simulink library "robotlib"  (R2025a)
settings: Solver=ode45  StartTime=0.0  StopTime=10.0  RelTol=1e-3  EnableMultiTasking=on
undefined symbols (not defined in the file): coder, Count, Data, Data_SL_Info, Datatype, Encoding, Encoding_SL_Info, Fields, Fields_SL_Info, Header, Height, Name, Name_SL_Info, Offset, PointStep, ros, RowStep, Step, Width
libraries: $bdroot x1
(part 1 of 2)
settings Model: Creator=The MathWorks, Inc.  LastModifiedBy=The MathWorks, Inc.
settings SolverCC: AlgebraicLoopSolver=TrustRegion  MaxZcPerStep=1.0
settings DataIOCC: LimitDataPoints=on  SaveFormat=Array  ReturnWorkspaceOutputs=off
settings OptimizationCC: ReuseModelBlockBuffer=off  LifeSpan=inf
settings DebuggingCC: SolverPrmCheckMsg=warning  UnconnectedInputMsg=warning  UnconnectedOutputMsg=warning  UnconnectedLineMsg=warning  AllowSymbolicDim=off  PregeneratedLibrarySubsystemCodeDiagnostic=none  SubsystemReferenceDiagnosticForUnitTest=warning  SFUnexpectedBacktrackingDiag=warning  SFNoUnconditionalDefaultTransitionDiag=warning  SFExecutionAtInitializationDiag=none  ArithmeticOperatorsInVariantConditions=warning
settings HardwareCC: ProdBitPerPointer=32.0  ProdBitPerSizeT=32.0  ProdBitPerPtrDiffT=32.0  ProdLargestAtomicFloat=None  ProdIntDivRoundTo=Undefined  ProdEndianess=Unspecified  ProdWordSize=32.0  ProdHWDeviceType=32-bit Generic
settings ModelReferenceCC: EnableRefExpFcnMdlSchedulingChecks=on  PropagateSignalLabelsOutOfModel=off
settings SFSimCC: SimUseLocalCustomCode=off
settings RTWCC: RTWUseLocalCustomCode=off  GPUComputeCapability=3.5  DLArmComputeVersion=19.05
settings CodeAppCC: StateflowObjectComments=on
settings GRTTargetCC: TargetLangStandard=C89/C90 (ANSI)
settings ConfigComp: CovScope=ReferencedModels  CovMetricSettings=dw  CovSaveCumulativeToWorkspaceVar=on  CovSaveSingleToWorkspaceVar=on  CovExternalEMLEnable=off  CovSFcnEnable=off

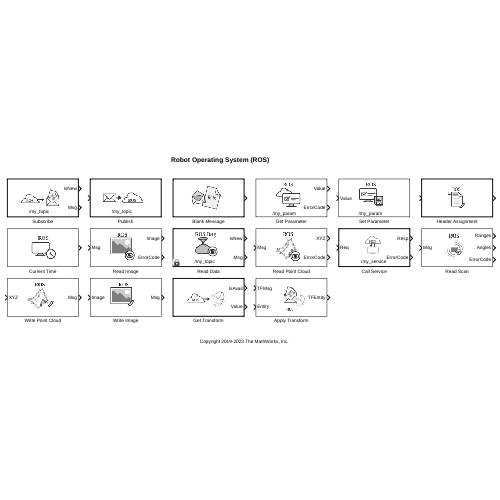
[thumbnail: Simulink's stored preview of the top-level diagram]
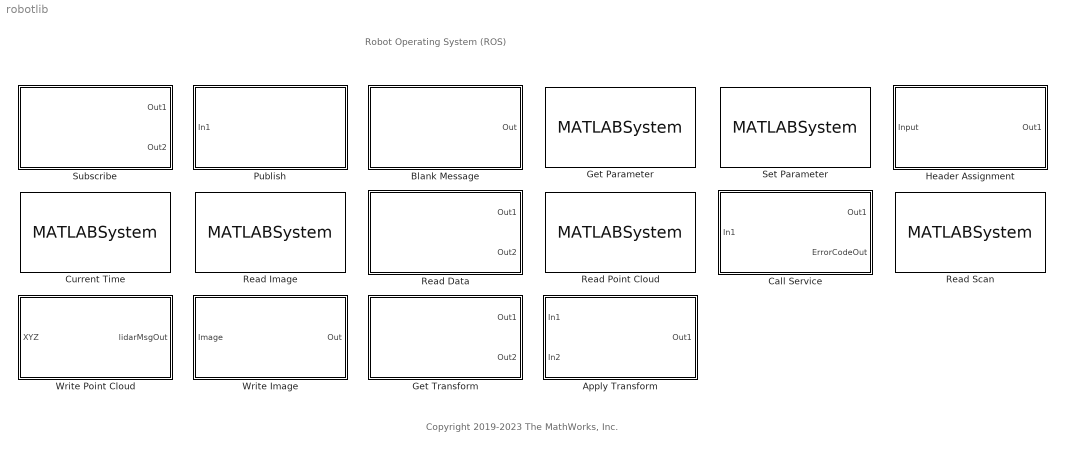
== system robotlib ==
  note: Copyright 2019-2023 The MathWorks, Inc.
  note: Robot Operating System (ROS)
  Apply Transform : Subsystem  InitFcn=ros.slros.internal.block.errorIfBlocksConflict(bdroot(gcb));  SystemSampleTime=SampleTime  mask(ros.slroscpp.internal.block.ApplyTransform){EntityMsgType=geometry_msgs/QuaternionStamped, SampleTime=-1}
      mask prompts: EntityMsgType "ros:slros:blockmask:EntityMsgPrompt"; SampleTime "Simulink:blkprm_prompts:AllBlksSampleTime"
      mask help: ros:slros:blockmask:ApplyTransformDescription
      mask init:
      | ros.slros.internal.block.ApplyTransformBlockMask.dispatch('maskInitialize', gcb);
      settings: ModelCloseFcn=ros.slros.internal.block.ApplyTransformBlockMask.dispatch('modelCloseFcn', gcb);
      mask Help: eval('ros.slros.internal.helpview(''rosApplyTransformBlock'')');
      mask TypeOptions EntityMsgType: ApplyTransform/EntityMsgType
      mask Callback EntityMsgType: ros.slros.internal.block.ApplyTransformBlockMask.dispatch('entityMsgTypeSelect', gcb);
      mask TypeOptions SampleTime: SystemSampleTime
      mask DialogControl DescGroupVar Prompt: ros:slros:blockmask:ApplyTransformMaskTitle
      mask DialogControl EntityMsgType Prompt: Entity message type:
      mask DialogControl SampleTime Prompt: Sample time (-1 for inherited):
      mask Display:
      | color('black');
      | port_label('input', 1, 'TFMsg');
      | port_label('input', 2, 'Entity');
      | port_label('output', 1, 'TFEntity');
  Blank Message : Subsystem  LoadFcn=ros.slros.internal.block.MessageBlockMask.dispatch('loadFcn', gcb);  InitFcn=ros.slros.internal.block.errorIfBlocksConflict(bdroot(gcb));  TreatAsAtomicUnit=on  mask(ROS Blank Message){messageClass=Message, entityType=geometry_msgs/Point, messageType=geometry_msgs/Point, SampleTime=inf, legacyBusStruct=off}
      mask prompts: messageClass "ros:slros:blockmask:MessageClassPrompt"; entityType "ros:slros:blockmask:TypePrompt"; messageType "ros:slros:blockmask:FullTypePrompt"; SampleTime "Simulink:blkprm_prompts:AllSrcBlksSampleTime"; legacyBusStruct "Use legacy bus structure"
      mask help: ros:slros:blockmask:BlankMsgDescription
      mask init:
      | ros.slros.internal.block.MessageBlockMask.dispatch('maskInitialize', gcb);
      settings: ModelCloseFcn=ros.slros.internal.block.MessageBlockMask.dispatch('modelCloseFcn', gcb);  PreSaveFcn=ros.slros.internal.block.MessageBlockMask.dispatch('preSaveFcn', gcb);
      mask Help: eval('ros.slros.internal.helpview(''rosBlankMsgBlock'')');
      mask TypeOptions messageClass: ros:slros:blockmask:MessageType_Msg | ros:slros:blockmask:MessageType_SrvReq | ros:slros:blockmask:MessageType_SrvResp
      mask Callback messageClass: ros.slros.internal.block.MessageBlockMask.dispatch('messageClassChange', gcb);
      mask Callback entityType: ros.slros.internal.block.MessageBlockMask.dispatch('entityTypeEdit', gcb);
      mask TypeOptions SampleTime: Constant/SampleTime
      mask DialogControl messageClass Prompt: Class:
      mask DialogControl entityType Prompt: Type:
      mask DialogControl id_msgTypeSelectBtn Prompt: ros:slros:blockmask:SelectPrompt
      mask DialogControl id_msgTypeSelectBtn Callback: ros.slros.internal.block.MessageBlockMask.dispatch('selectButtonPressed', gcb);
      mask DialogControl messageType Prompt: Fully resolved type:
      mask DialogControl SampleTime Prompt: Sample time:
      mask Display: color('black');
  Call Service : Subsystem  InitFcn=ros.slros.internal.block.errorIfBlocksConflict(bdroot(gcb));  TreatAsAtomicUnit=on  mask(ROS Call Service){topicSource=Select from ROS network, service=/my_service, serviceType=std_srvs/Empty, connectionTimeout=5, keepPersistent=off, ShowErrorCodeOutput=on, outputStreamWsVar=, legacyBusStruct=off}
      mask prompts: topicSource "ros:slros:svccaller:SourcePrompt"; service "ros:slros:svccaller:NamePrompt"; serviceType "ros:slros:svccaller:TypePrompt"; connectionTimeout "ros:slros:svccaller:ConnectionTimeoutPrompt"; keepPersistent "ros:slros:svccaller:KeepPersistentPrompt"; ShowErrorCodeOutput "ros:slros:blockmask:ShowErrorCodePrompt"; outputStreamWsVar "ros:slros:blockmask:WorkspaceStreamPrompt"; legacyBusStruct "Use legacy bus structure"
      mask help: ros:slros:svccaller:MaskDescription
      mask init:
      | ros.slros.internal.block.ServiceCallBlockMask.dispatch('maskInitialize', gcb);
      settings: ModelCloseFcn=ros.slros.internal.block.ServiceCallBlockMask.dispatch('modelCloseFcn', gcb);
      mask Help: eval('ros.slros.internal.helpview(''rosCallServiceBlock'')');
      mask TypeOptions topicSource: ros:slros:blockmask:TopicSourceFromNetwork | ros:slros:blockmask:TopicSourceSpecifyOwn
      mask Callback topicSource: ros.slros.internal.block.ServiceCallBlockMask.dispatch('serviceSourceSelect', gcb);
      mask Callback service: ros.slros.internal.block.ServiceCallBlockMask.dispatch('serviceEdit', gcb);
      mask Callback connectionTimeout: ros.slros.internal.block.ServiceCallBlockMask.dispatch('connectionTimeoutEdit', gcb);
      mask Callback keepPersistent: ros.slros.internal.block.ServiceCallBlockMask.dispatch('updateSubsystem', gcb);
      mask TypeOptions outputStreamWsVar: ServiceCaller/OutputStreamWsVar
      mask DialogControl id_netAddrLink Prompt: ros:slros:blockmask:ConfigNetworkAddrLinkText
      mask DialogControl id_netAddrLink Callback: ros.slros.internal.block.ServiceCallBlockMask.dispatch('configureNetworkAddrDlg', gcb);
      mask DialogControl serviceGroup Prompt: Service
      mask DialogControl topicSource Prompt: Source:
      mask DialogControl service Prompt: Name:
      mask DialogControl id_topicSelectBtn Prompt: ros:slros:blockmask:SelectPrompt
      mask DialogControl id_topicSelectBtn Callback: ros.slros.internal.block.ServiceCallBlockMask.dispatch('serviceSelect', gcb, 'ros.slros.internal.dlg.ServiceSelector');
      mask DialogControl serviceType Prompt: Type:
      mask DialogControl id_msgTypeSelectBtn Prompt: ros:slros:blockmask:SelectPrompt
      mask DialogControl id_msgTypeSelectBtn Callback: ros.slros.internal.block.ServiceCallBlockMask.dispatch('serviceTypeSelect', gcb, 'ros.slros.internal.dlg.ServiceTypeSelector');
      mask DialogControl connectionTimeout Prompt: Connection timeout:
      mask DialogControl keepPersistent Prompt: Keep persistent connection
      mask DialogControl ShowErrorCodeOutput Prompt: Show ErrorCode output port
      mask DialogControl outputStreamWsVar Prompt: Workspace stream:
      mask Display:
      | color('black');
      | text(0.5, 0.15, '/my_service', 'horizontalAlignment', 'center');
      | port_label('input', 1, 'Req');
      | port_label('output', 1, 'Resp');
      | port_label('output', 2, 'ErrorCode');
  Current Time : MATLABSystem  InitFcn=ros.slros.internal.block.CurrentTimeBlockMask.dispatch('initFcn', gcb);  System=ros.slros.internal.block.CurrentTime  OutputFormat=bus  SampleTime=SampleTime  ModelName=robotlib  mask(ros.slros.internal.block.CurrentTime){OutputFormat=bus, SampleTime=-1, StreamWSVar=, ModelName=robotlib}
      mask prompts: OutputFormat "ros:slros:rostime:OutputFormatPrompt"; SampleTime "ros:slros:blockmask:SampleTimePrompt"; StreamWSVar "ros:slros:blockmask:WorkspaceStreamPrompt"; ModelName "ros:slros:blockmask:ModelNamePrompt"
      mask help: ros:slros:rostime:MaskDescription
      mask init:
      | ros.slros.internal.block.CurrentTimeBlockMask.dispatch('maskInitialize', gcb);
      settings: ModelCloseFcn=ros.slros.internal.block.CurrentTimeBlockMask.dispatch('modelCloseFcn', gcb);
      mask Help: eval('ros.slros.internal.helpview(''rosCurrentTimeBlock'')');
      mask TypeOptions OutputFormat: OutputFormat
      mask TypeOptions SampleTime: SampleTime
      mask TypeOptions StreamWSVar: StreamWSVar
      mask TypeOptions ModelName: ModelName
      mask DialogControl DescGroupVar Prompt: ros:slros:rostime:MaskTitle
      mask DialogControl OutputFormat Prompt: Output format:
      mask DialogControl SampleTime Prompt: Sample time:
      mask DialogControl StreamWSVar Prompt: Workspace stream:
      mask DialogControl ModelName Prompt: Model name:
      mask Display: color('black');
  Get Parameter : MATLABSystem  System=ros.slros.internal.block.GetParameter  ParameterSource=Select from ROS network  ParameterName=/my_param  ParameterType=double  ParameterMaxArrayLength=ParameterMaxArrayLength  ParameterInitialValue=ParameterInitialValue  ShowErrorCodeOutput=on  SampleTime=SampleTime  ModelName=robotlib  BlockId=ParamGet_robotlib_148  mask(ROS Get Parameter){ParameterSource=Select from ROS network, ParameterName=/my_param, ParameterType=double, ParameterMaxArrayLength=16, ParameterInitialValue=0.0, SampleTime=-1, ShowErrorCodeOutput=on, ModelName=robotlib, BlockId=ParamGet_robotlib_148}
      mask prompts: ParameterSource "ros:slros:blockmask:ParameterSourcePrompt"; ParameterName "ros:slros:blockmask:ParameterNamePrompt"; ParameterType "ros:slros:blockmask:ParameterDataTypePrompt"; ParameterMaxArrayLength "Maximum length:"; ParameterInitialValue "ros:slros:blockmask:ParameterInitialValuePrompt"; SampleTime "ros:slros:blockmask:SampleTimePrompt"; ShowErrorCodeOutput "ros:slros:blockmask:ShowErrorCodePrompt"; ModelName "Name of Simulink model:"; BlockId "Simulink Block Identifier:"
      mask help: ros:slros:blockmask:GetParameterDescription
      mask init:
      | ros.slros.internal.block.GetParameterBlockMask.dispatch('maskInitialize',gcb);
      mask Help: eval('ros.slros.internal.helpview(''rosGetParameterBlock'')');
      mask TypeOptions ParameterSource: ParameterSource
      mask Callback ParameterSource: ros.slros.internal.block.GetParameterBlockMask.dispatch('setParameterSource', gcb);
      mask TypeOptions ParameterName: ParameterName
      mask TypeOptions ParameterType: ParameterType
      mask Callback ParameterType: ros.slros.internal.block.GetParameterBlockMask.dispatch('setParameterType', gcb);
      mask TypeOptions ParameterMaxArrayLength: ParameterMaxArrayLength
      mask TypeOptions ParameterInitialValue: ParameterInitialValue
      mask TypeOptions SampleTime: SampleTime
      mask TypeOptions ShowErrorCodeOutput: ShowErrorCodeOutput
      mask TypeOptions ModelName: ModelName
      mask TypeOptions BlockId: BlockId
      mask DialogControl DescGroupVar Prompt: ros:slros:blockmask:GetParameterTitle
      mask DialogControl id_netAddrLink Prompt: ros:slros:blockmask:ConfigNetworkAddrLinkText
      mask DialogControl id_netAddrLink Callback: ros.slros.internal.block.GetParameterBlockMask.dispatch('configureNetworkAddrDlg', gcb);
      mask DialogControl ROSParameterContainer Prompt: ros:slros:blockmask:ROSParameterPrompt
      mask DialogControl ParameterSource Prompt: Source:
      mask DialogControl ParameterName Prompt: Name:
      mask DialogControl SelectCallback Prompt: ros:slros:blockmask:SelectPrompt
      mask DialogControl SelectCallback Callback: ros.slros.internal.block.GetParameterBlockMask.dispatch('onSelectFromNetwork', gcb);
      mask DialogControl ParameterType Prompt: Data type:
      mask DialogControl ParameterInitialValue Prompt: Initial value:
      mask DialogControl SampleTime Prompt: Sample time:
      mask DialogControl ShowErrorCodeOutput Prompt: Show ErrorCode output port
  Get Transform : Subsystem  InitFcn=ros.slros.internal.block.errorIfBlocksConflict(bdroot(gcb));  TreatAsAtomicUnit=on  mask(ros.slroscpp.internal.block.GetTransform){FrameSource=Select from ROS network, TargetFrame=, SourceFrame=, OutputFormat=bus, SampleTime=-1}
      mask prompts: FrameSource "ros:slros:blockmask:FrameSourcePrompt"; TargetFrame "ros:slros:blockmask:TargetPrompt"; SourceFrame "ros:slros:blockmask:SourcePrompt"; OutputFormat "ros:slros:blockmask:OutputFormatPrompt"; SampleTime "Simulink:blkprm_prompts:AllSrcBlksSampleTime"
      mask help: ros:slros:blockmask:GetTransformDescription
      mask init:
      | ros.slros.internal.block.GetTransformBlockMask.dispatch('maskInitialize',gcb);
      settings: ModelCloseFcn=ros.slros.internal.block.GetTransformBlockMask.dispatch('modelCloseFcn', gcb);
      mask Help: eval('ros.slros.internal.helpview(''rosGetTransformBlock'')');
      mask TypeOptions FrameSource: ros:slros:blockmask:TopicSourceFromNetwork | ros:slros:blockmask:TopicSourceSpecifyOwn
      mask Callback FrameSource: ros.slros.internal.block.GetTransformBlockMask.dispatch('frameSourceSelect',gcb);
      mask TypeOptions TargetFrame: SourceBlock/TargetFrame
      mask TypeOptions SourceFrame: SourceBlock/SourceFrame
      mask TypeOptions OutputFormat: SourceBlock/OutputFormat
      mask TypeOptions SampleTime: Constant/SampleTime
      mask DialogControl DescGroupVar Prompt: ros:slros:blockmask:GetTransformMaskTitle
      mask DialogControl Container4 Prompt: Main
      mask DialogControl FrameSource Prompt: Frame source:
      mask DialogControl TargetFrame Prompt: Target:
      mask DialogControl id_targetSelectBtn Prompt: ros:slros:blockmask:SelectPrompt
      mask DialogControl id_targetSelectBtn Callback: ros.slros.internal.block.GetTransformBlockMask.dispatch('frameSelect',gcb,'TargetFrame','ros.slros.internal.dlg.FrameSelector');
      mask DialogControl SourceFrame Prompt: Source:
      mask DialogControl id_sourceSelectBtn Prompt: ros:slros:blockmask:SelectPrompt
      mask DialogControl id_sourceSelectBtn Callback: ros.slros.internal.block.GetTransformBlockMask.dispatch('frameSelect',gcb,'SourceFrame','ros.slros.internal.dlg.FrameSelector');
      mask DialogControl OutputFormat Prompt: Output format:
      mask DialogControl SampleTime Prompt: Sample time:
      mask Display:
      | color('black');
      | port_label('output', 1, 'IsAvail');
      | port_label('output', 2, 'Value');
  Header Assignment : Subsystem  TreatAsAtomicUnit=on  mask(ROS Header){SetFrameID=off, FrameID=, InsertTimeStamp=off, SetHeaderFieldName=Use the default Header field name, HeaderFieldName=Header}
      mask prompts: SetFrameID "ros:slros:blockmask:SetFrameIdPrompt"; InsertTimeStamp "ros:slros:blockmask:SetTimestampPrompt"; SetHeaderFieldName "ros:slros:blockmask:SetHdrFldNamePrompt"
      mask help: ros:slros:blockmask:HdrAssignDescription
      mask init:
      | ros.slros.internal.block.HeaderAssignmentBlockMask.dispatch('maskInitialize', gcb);
      mask Help: eval('ros.slros.internal.helpview(''rosHeaderAssignment'')');
      mask Callback SetFrameID: ros.slros.internal.block.HeaderAssignmentBlockMask.dispatch('checkSetFrameId', gcb);
      mask Callback FrameID: ros.slros.internal.block.HeaderAssignmentBlockMask.dispatch('setFrameId', gcb);
      mask TypeOptions SetHeaderFieldName: ros:slros:blockmask:HdrFldNameDefault | ros:slros:blockmask:HdrFldNameSpecifyOwn
      mask Callback SetHeaderFieldName: ros.slros.internal.block.HeaderAssignmentBlockMask.dispatch('checkSetHeaderFieldName', gcb);
      mask Callback HeaderFieldName: ros.slros.internal.block.HeaderAssignmentBlockMask.dispatch('setHeaderFieldName', gcb);
      mask DialogControl SetFrameID Prompt: Set Frame ID:
      mask DialogControl InsertTimeStamp Prompt: Set Timestamp
      mask DialogControl SetHeaderFieldName Prompt: Header field name:
      mask Display:
      | color('white');
      | 
      | plot([100,100,100,100],[100,100,100,100]);
      | 
      | plot([0,0,0,0],[0,0,0,0]);
  Publish : Subsystem  InitFcn=ros.slros.internal.block.errorIfBlocksConflict(bdroot(gcb));  TreatAsAtomicUnit=on  mask(ROS Publish){topicSource=Select from ROS network, topic=/my_topic, messageType=geometry_msgs/Point, OutputStreamWsVar=, legacyBusStruct=off, messageQueueLength=1}
      mask prompts: topicSource "ros:slros:blockmask:TopicSourcePrompt"; topic "ros:slros:blockmask:TopicPrompt"; messageType "ros:slros:blockmask:MessageTypePrompt"; OutputStreamWsVar "ros:slros:blockmask:PublisherOutputStreamPrompt"; legacyBusStruct "Use legacy bus structure"; messageQueueLength "ros:slros:blockmask:PublisherMsgQueuePrompt"
      mask help: ros:slros:blockmask:PublisherDescription
      mask init:
      | ros.slros.internal.block.PublishBlockMask.dispatch('maskInitialize', gcb);
      settings: ModelCloseFcn=ros.slros.internal.block.PublishBlockMask.dispatch('modelCloseFcn', gcb);
      mask Help: eval('ros.slros.internal.helpview(''rosPublishBlock'')');
      mask TypeOptions topicSource: ros:slros:blockmask:TopicSourceFromNetwork | ros:slros:blockmask:TopicSourceSpecifyOwn
      mask Callback topicSource: ros.slros.internal.block.PublishBlockMask.dispatch('topicSourceSelect', gcb);
      mask Callback topic: ros.slros.internal.block.PublishBlockMask.dispatch('topicEdit', gcb);
      mask TypeOptions OutputStreamWsVar: SinkBlock/OutputStreamWsVar
      mask TypeOptions messageQueueLength: SinkBlock/MessageQueueLen
      mask DialogControl id_netAddrLink Prompt: ros:slros:blockmask:ConfigNetworkAddrLinkText
      mask DialogControl id_netAddrLink Callback: ros.slros.internal.block.PublishBlockMask.dispatch('configureNetworkAddrDlg', gcb);
      mask DialogControl Container13 Prompt: Main
      mask DialogControl topicSource Prompt: Topic source:
      mask DialogControl topic Prompt: Topic:
      mask DialogControl id_topicSelectBtn Prompt: ros:slros:blockmask:SelectPrompt
      mask DialogControl id_topicSelectBtn Callback: ros.slros.internal.block.PublishBlockMask.dispatch('topicSelect', gcb, 'ros.slros.internal.dlg.TopicSelector');
      mask DialogControl messageType Prompt: Message type:
      mask DialogControl id_msgTypeSelectBtn Prompt: ros:slros:blockmask:SelectPrompt
      mask DialogControl id_msgTypeSelectBtn Callback: ros.slros.internal.block.PublishBlockMask.dispatch('messageTypeSelect', gcb, 'ros.slros.internal.dlg.MessageTypeSelector');
      mask DialogControl OutputStreamWsVar Prompt: Output stream workspace variable:
      mask DialogControl id_cgContainer Prompt: ros:slros:blockmask:CodeGenTabTitle
      mask DialogControl messageQueueLength Prompt: Length of publish queue:
      mask Display:
      | color('black');
      | text(0.45, 0.15, '/my_topic', 'horizontalAlignment', 'center');
  Read Data : Subsystem  InitFcn=ros.slros.internal.block.errorIfBlocksConflict(bdroot(gcb));  TreatAsAtomicUnit=on  mask(Read Data from ROS Bag){topic=/my_topic, sampleTime=-1, logfileType=rosbag, modelName=robotlib, msgType=}
      mask prompts: topic "ros:slros:readlog:TopicPrompt"; sampleTime "ros:slros:readlog:SampleTimePrompt"
      mask help: ros:slros:readlog:ReadDataDescription
      mask init:
      | ros.slros.internal.block.ReadDataBlockMask.blockInitFcn(gcb);
      settings: ModelCloseFcn=ros.slros.internal.block.ReadDataBlockMask.modelCloseFcn(gcb);
      mask Help: eval('ros.slros.internal.helpview(''rosReadDataBlock'')');
      mask TypeOptions topic: SourceBlock/Topic
      mask TypeOptions sampleTime: SourceBlock/SampleTime
      mask TypeOptions logfileType: SourceBlock/LogfileType
      mask TypeOptions modelName: SourceBlock/ModelName
      mask TypeOptions msgType: SourceBlock/MsgType
      mask DialogControl id_logDataLink Prompt: ros:slros:readlog:LoadDataPrompt
      mask DialogControl id_logDataLink Callback: ros.slros.internal.block.ReadDataBlockMask.loadLogfileLink(gcb)
      mask DialogControl topic Prompt: Topic:
      mask DialogControl id_topicSelectBtn Prompt: ros:slros:readlog:SelectPrompt
      mask DialogControl id_topicSelectBtn Callback: ros.slros.internal.block.ReadDataBlockMask.topicSelectButton(gcb)
      mask DialogControl sampleTime Prompt: Sample time:
      mask Display:
      | color('black');
      | text(0.45, 0.15, '/my_topic', 'horizontalAlignment', 'center');
      | port_label('output', 1, 'IsNew');
      | port_label('output', 2, 'Msg');
  Read Image : MATLABSystem  InitFcn=ros.slros.internal.block.errorIfBlocksConflict(bdroot(gcb));  System=ros.slros.internal.block.ReadImage  MaximumImageSize=[ 2000, 2000 ]  ImageEncoding=rgb8  ShowAlphaOutput=off  ShowErrorCodeOutput=on  VariableSizeOutputs=off
      mask Type: ros.slros.internal.block.ReadImage
  Read Point Cloud : MATLABSystem  InitFcn=ros.slros.internal.block.errorIfBlocksConflict(bdroot(gcb));  System=ros.slros.internal.block.ReadPointCloud  MaximumPointCloudSize=[ 480, 640 ]  PreserveStructure=off  ShowRGBOutput=off  ShowIntensityOutput=off  ShowErrorCodeOutput=on  VariableSizeOutputs=off
      mask Type: ros.slros.internal.block.ReadPointCloud
  Read Scan : MATLABSystem  InitFcn=ros.slros.internal.block.errorIfBlocksConflict(bdroot(gcb));  System=ros.slros.internal.block.ReadScan  MaximumArrayLength=100  ShowAnglesOutput=on  ShowIntensityOutput=off  ShowErrorCodeOutput=on  VariableSizeOutputs=off
      mask Type: ros.slros.internal.block.ReadScan
  Set Parameter : MATLABSystem  System=ros.slros.internal.block.SetParameter  ParameterSource=Select from ROS network  ParameterName=/my_param  ParameterType=double  ModelName=robotlib  BlockId=ParamSet_robotlib_107  mask(ROS Set Parameter){ParameterSource=Select from ROS network, ParameterName=/my_param, ParameterType=double, ModelName=robotlib, BlockId=ParamSet_robotlib_107}
      mask prompts: ParameterSource "ros:slros:blockmask:ParameterSourcePrompt"; ParameterName "ros:slros:blockmask:ParameterNamePrompt"; ParameterType "ros:slros:blockmask:ParameterDataTypePrompt"; ModelName "Name of Simulink model:"; BlockId "Simulink Block Identifier:"
      mask help: ros:slros:blockmask:SetParameterDescription
      mask init:
      | ros.slros.internal.block.SetParameterBlockMask.dispatch('maskInitialize',gcb);
      mask Help: eval('ros.slros.internal.helpview(''rosSetParameterBlock'')');
      mask TypeOptions ParameterSource: ParameterSource
      mask Callback ParameterSource: ros.slros.internal.block.SetParameterBlockMask.dispatch('setParameterSource', gcb);
      mask TypeOptions ParameterName: ParameterName
      mask TypeOptions ParameterType: ParameterType
      mask TypeOptions ModelName: ModelName
      mask TypeOptions BlockId: BlockId
      mask DialogControl DescGroupVar Prompt: ros:slros:blockmask:SetParameterTitle
      mask DialogControl id_netAddrLink Prompt: ros:slros:blockmask:ConfigNetworkAddrLinkText
      mask DialogControl id_netAddrLink Callback: ros.slros.internal.block.SetParameterBlockMask.dispatch('configureNetworkAddrDlg', gcb);
      mask DialogControl ROSParameterContainer Prompt: ros:slros:blockmask:ROSParameterPrompt
      mask DialogControl ParameterSource Prompt: Source:
      mask DialogControl ParameterName Prompt: Name:
      mask DialogControl SelectCallback Prompt: ros:slros:blockmask:SelectPrompt
      mask DialogControl SelectCallback Callback: ros.slros.internal.block.SetParameterBlockMask.dispatch('onSelectFromNetwork', gcb);
      mask DialogControl ParameterType Prompt: Data type:
  Subscribe : Subsystem  InitFcn=ros.slros.internal.block.errorIfBlocksConflict(bdroot(gcb));  TreatAsAtomicUnit=on  mask(ROS Subscribe){topicSource=Select from ROS network, topic=/my_topic, messageType=geometry_msgs/Point, SampleTime=-1, InputStreamWsVar=, legacyBusStruct=off, messageQueueLength=1}
      mask prompts: topicSource "ros:slros:blockmask:TopicSourcePrompt"; topic "ros:slros:blockmask:TopicPrompt"; messageType "ros:slros:blockmask:MessageTypePrompt"; SampleTime "ros:slros:blockmask:SampleTimePrompt"; InputStreamWsVar "ros:slros:blockmask:SubscriberInputStreamPrompt"; legacyBusStruct "Use legacy bus structure"; messageQueueLength "ros:slros:blockmask:SubscriberMsgQueuePrompt"
      mask help: ros:slros:blockmask:SubscriberDescription
      mask init:
      | ros.slros.internal.block.SubscribeBlockMask.dispatch('maskInitialize', gcb);
      settings: ModelCloseFcn=ros.slros.internal.block.SubscribeBlockMask.dispatch('modelCloseFcn', gcb);
      mask Help: eval('ros.slros.internal.helpview(''rosSubscribeBlock'')');
      mask TypeOptions topicSource: ros:slros:blockmask:TopicSourceFromNetwork | ros:slros:blockmask:TopicSourceSpecifyOwn
      mask Callback topicSource: ros.slros.internal.block.SubscribeBlockMask.dispatch('topicSourceSelect', gcb);
      mask Callback topic: ros.slros.internal.block.SubscribeBlockMask.dispatch('topicEdit', gcb);
      mask TypeOptions SampleTime: Constant/SampleTime
      mask TypeOptions InputStreamWsVar: SourceBlock/InputStreamWsVar
      mask TypeOptions messageQueueLength: SourceBlock/MessageQueueLen
      mask DialogControl id_netAddrLink Prompt: ros:slros:blockmask:ConfigNetworkAddrLinkText
      mask DialogControl id_netAddrLink Callback: ros.slros.internal.block.SubscribeBlockMask.dispatch('configureNetworkAddrDlg', gcb);
      mask DialogControl Container13 Prompt: Main
      mask DialogControl topicSource Prompt: Topic source:
      mask DialogControl topic Prompt: Topic:
      mask DialogControl id_topicSelectBtn Prompt: ros:slros:blockmask:SelectPrompt
      mask DialogControl id_topicSelectBtn Callback: ros.slros.internal.block.SubscribeBlockMask.dispatch('topicSelect', gcb, 'ros.slros.internal.dlg.TopicSelector');
      mask DialogControl messageType Prompt: Message type:
      mask DialogControl id_msgTypeSelectBtn Prompt: ros:slros:blockmask:SelectPrompt
      mask DialogControl id_msgTypeSelectBtn Callback: ros.slros.internal.block.SubscribeBlockMask.dispatch('messageTypeSelect', gcb, 'ros.slros.internal.dlg.MessageTypeSelector');
      mask DialogControl SampleTime Prompt: Sample time:
      mask DialogControl InputStreamWsVar Prompt: Input stream workspace variable:
      mask DialogControl id_cgContainer Prompt: ros:slros:blockmask:CodeGenTabTitle
      mask DialogControl messageQueueLength Prompt: Length of subscribe callback queue:
      mask Display:
      | color('black');
      | text(0.45, 0.15, '/my_topic', 'horizontalAlignment', 'center');
      | port_label('output', 1, 'IsNew');
      | port_label('output', 2, 'Msg');
  Write Image : Subsystem  InitFcn=|  mask(ROS Write Image){ImageEncoding=rgb8, EncodingStruct=ros.msg.sensor_msgs.internal.ImageEncoding.info(coder.const('rgb8')), HasAlpha=off, messageType=sensor_msgs/Image}
      | ros.slros.internal.block.errorIfBlocksConflict(bdroot(gcb));
      | ros.slros.internal.block.WriteImageBlockMask.dispatch('maskInitialize', gcb);
      mask prompts: ImageEncoding "ros:slros:blockmask:ImageEncodingPrompt"
      mask init:
      | ros.slros.internal.block.WriteImageBlockMask.dispatch('maskInitialize', gcb);
      mask Help: eval('ros.slros.internal.helpview(''rosWriteImBlock'')');
      mask TypeOptions ImageEncoding: rgb8 | rgba8 | rgb16 | rgba16 | bgr8 | bgra8 | bgr16 | bgra16 | mono8 | mono16 | 32fc1 | 32fc2 | 32fc3 | 32fc4 | 64fc1 | 64fc2 | 64fc3 | 64fc4 | 8uc1 | 8uc2 | 8uc3 | 8uc4 | 8sc1 | 8sc2 | 8sc3 | 8sc4 | 16uc1 | 16uc2 | 16uc3 | 16uc4 | 16sc1 | 16sc2 | 16sc3 | 16sc4 | 32sc1 | 32sc2 | 32sc3 | 32sc4
      mask DialogControl DescGroupVar Prompt: ros:slros:blockmask:WriteImageTitle
      mask DialogControl DescTextVar Prompt: ros:slros:blockmask:WriteImageDescription
      mask DialogControl Settings Prompt: ros:slros:blockmask:ImagePropertiesPrompt
      mask DialogControl ImageEncoding Prompt: Image encoding:
      mask Display: port_label('input',1,'Image');port_label('output',1,'Msg');
  Write Point Cloud : Subsystem  InitFcn=|  mask(ROS Write Point Cloud){messageType=sensor_msgs/PointCloud2, Encoding=none, HasRGB=false, HasAlpha=false, HasIntensityCheck=off, HasIntensity=false, FieldNamesStruct=struct('x', 'single', 'y', 'single', 'z', 'single')}
      | ros.slros.internal.block.errorIfBlocksConflict(bdroot(gcb));
      | ros.slros.internal.block.WritePointCloudBlockMask.dispatch('maskInitialize', gcb);
      mask prompts: Encoding "ros:slros:blockmask:SelectRGBInputPrompt"; HasIntensityCheck "ros:slros:blockmask:WriteIntensityFieldPrompt"
      mask init:
      | ros.slros.internal.block.WritePointCloudBlockMask.dispatch('maskInitialize', gcb);
      mask Help: eval('ros.slros.internal.helpview(''rosWritePCBlock'')');
      mask TypeOptions Encoding: none | rgb | rgba
      mask DialogControl DescGroupVar Prompt: ros:slros:blockmask:WritePointCloudTitle
      mask DialogControl DescTextVar Prompt: ros:slros:blockmask:WritePointCloudDescription
      mask DialogControl ParameterGroupVar Prompt: ros:slros:blockmask:InputConfiguration
      mask DialogControl Encoding Prompt: Select color field
      mask DialogControl HasIntensityCheck Prompt: Write to Intensity field
      mask Display: port_label('input', 1, 'XYZ'); port_label('output', 1, 'Msg');

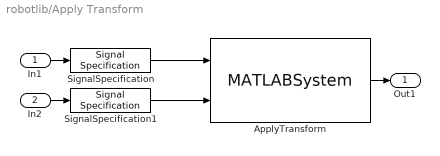
== system robotlib/Apply Transform ==
  In1 : Inport
  In2 : Inport  Port=2
  ApplyTransform : MATLABSystem  System=ros.slroscpp.internal.block.ApplyTransform  EntityMsgType=geometry_msgs/QuaternionStamped  ModelName=robotlib  BlockId=APTF_robotlib_180  SLOutputBusName=SL_Bus_robotlib_geometry_msgs_QuaternionStamped
      mask Type: ros.slroscpp.internal.block.ApplyTransform
  SignalSpecification : SignalSpecification  OutDataTypeStr=Bus: SL_Bus_robotlib_geometry_msgs_TransformStamped  BusOutputAsStruct=on
      settings: LockScale=on
  SignalSpecification1 : SignalSpecification  OutDataTypeStr=Bus: SL_Bus_robotlib_geometry_msgs_QuaternionStamped  BusOutputAsStruct=on
      settings: LockScale=on
  Out1 : Outport
  wires:
  ApplyTransform/1 -> Out1/1
  In1/1 -> SignalSpecification/1
  SignalSpecification/1 -> ApplyTransform/1
  In2/1 -> SignalSpecification1/1
  SignalSpecification1/1 -> ApplyTransform/2

== system robotlib/Blank Message ==
  Constant : Constant  InitFcn=ros.slros.internal.block.MessageBlockMask.dispatch('constantBlkInitFcn', gcb);  Value=0  OutDataTypeStr=Bus: SL_Bus_robotlib_geometry_msgs_Point  SampleTime=SampleTime  LockScale=on
  Out : Outport  VectorParamsAs1DForOutWhenUnconnected=off  LockScale=on
  wires:
  Constant/1 -> Out/1

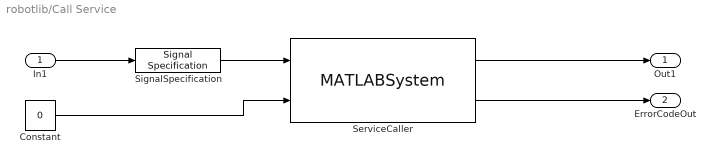
== system robotlib/Call Service ==
  In1 : Inport  LockScale=on
  Constant : Constant  InitFcn=ros.slros.internal.block.ServiceCallBlockMask.dispatch('constantBlkInitFcn', gcb);  Value=0  VectorParams1D=off  OutDataTypeStr=Bus: SL_Bus_robotlib_std_srvs_EmptyResponse  SampleTime=-1  LockScale=on
  ServiceCaller : MATLABSystem  InitFcn=ros.slros.internal.block.ServiceCallBlockMask.dispatch('sysobjInitFcn', gcb);  System=ros.slroscpp.internal.block.ServiceCaller  ServiceName=/my_service  ServiceType=std_srvs/Empty  ConnectionTimeout=5  IsPersistentConnection=off  ModelName=untitled  BlockId=serv1
      mask Type: ros.slroscpp.internal.block.ServiceCaller
  SignalSpecification : SignalSpecification  OutDataTypeStr=Bus: SL_Bus_robotlib_std_srvs_EmptyRequest  BusOutputAsStruct=on
      settings: LockScale=on
  Out1 : Outport  VectorParamsAs1DForOutWhenUnconnected=off
  ErrorCodeOut : Outport  Port=2  VectorParamsAs1DForOutWhenUnconnected=off
  wires:
  ServiceCaller/1 -> Out1/1
  In1/1 -> SignalSpecification/1
  SignalSpecification/1 -> ServiceCaller/1
  Constant/1 -> ServiceCaller/2
  ServiceCaller/2 -> ErrorCodeOut/1

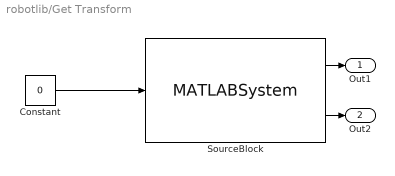
== system robotlib/Get Transform ==
  Constant : Constant  Value=0  VectorParams1D=off  OutDataTypeStr=Bus: SL_Bus_robotlib_geometry_msgs_TransformStamped  SampleTime=SampleTime  LockScale=on
  SourceBlock : MATLABSystem  System=ros.slroscpp.internal.block.GetTransform  SLBusName=SL_Bus_robotlib_geometry_msgs_TransformStamped  OutputFormat=bus  SampleTime=-1  ModelName=robotlib  BlockId=TF_robotlib_175
      mask Type: ros.slroscpp.internal.block.GetTransform
  Out1 : Outport
  Out2 : Outport  Port=2
  wires:
  Constant/1 -> SourceBlock/1
  SourceBlock/1 -> Out1/1
  SourceBlock/2 -> Out2/1

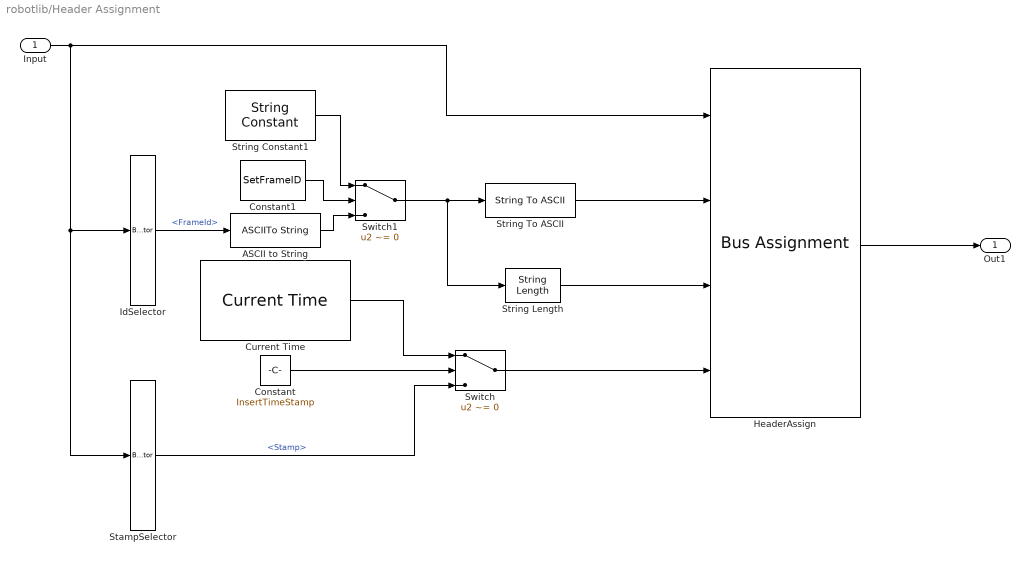
== system robotlib/Header Assignment ==
  Input : Inport
  ASCII to String : ASCIIToString
  Constant : Constant  Value=InsertTimeStamp
  Constant1 : Constant  Value=SetFrameID
  Current Time : $bdroot/Current Time  OutputFormat=bus  SampleTime=-1  ModelName=mNewHeaderAssignmentLogging
  HeaderAssign : BusAssignment  AssignedSignals=Header.FrameId,Header.FrameId_SL_Info.CurrentLength,Header.Stamp
  IdSelector : BusSelector  OutputSignals=Header.FrameId
  StampSelector : BusSelector  OutputSignals=Header.Stamp
  String Constant1 : StringConstant  String=FrameID
  String Length : StringLength
  String To ASCII : StringToASCII  OutputVectorSize=128
  Switch : Switch  Criteria=u2 ~= 0  Threshold=1.5  SaturateOnIntegerOverflow=off  InputSameDT=off
  Switch1 : Switch  Criteria=u2 ~= 0  Threshold=1.5  SaturateOnIntegerOverflow=off  InputSameDT=off
  Out1 : Outport
  wires:
  Switch1/1 -> String Length/1, String To ASCII/1
  String To ASCII/1 -> HeaderAssign/2
  HeaderAssign/1 -> Out1/1
  String Length/1 -> HeaderAssign/3
  Switch/1 -> HeaderAssign/4
  Constant/1 -> Switch/2
  Input/1 -> StampSelector/1, IdSelector/1, HeaderAssign/1
  StampSelector/1 -> Switch/3  "<Stamp>"
  Constant1/1 -> Switch1/2
  String Constant1/1 -> Switch1/1
  ASCII to String/1 -> Switch1/3
  IdSelector/1 -> ASCII to String/1  "<FrameId>"
  Current Time/1 -> Switch/1

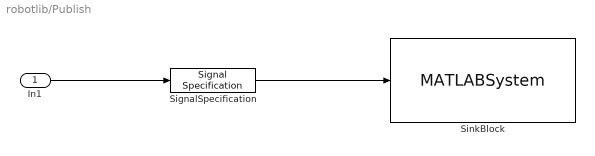
== system robotlib/Publish ==
  In1 : Inport  LockScale=on
  SignalSpecification : SignalSpecification  OutDataTypeStr=Bus: SL_Bus_robotlib_geometry_msgs_Point  BusOutputAsStruct=on
      settings: LockScale=on
  SinkBlock : MATLABSystem  System=ros.slroscpp.internal.block.Publisher  MessageQueueLen=messageQueueLength  ROSTopic=/my_topic  ROSMessageType=geometry_msgs/Point  SLBusName=SL_Bus_robotlib_geometry_msgs_Point  ModelName=robotlib  BlockId=Pub_robotlib_94
      mask Type: ros.slroscpp.internal.block.Publisher
  wires:
  In1/1 -> SignalSpecification/1
  SignalSpecification/1 -> SinkBlock/1

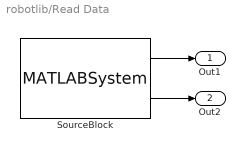
== system robotlib/Read Data ==
  SourceBlock : MATLABSystem  System=ros.slros.internal.block.ReadData  LogfileType=rosbag  Topic=/my_topic  SampleTime=sampleTime  ModelName=robotlib
      mask Type: ros.slros.internal.block.ReadData
  Out1 : Outport  VectorParamsAs1DForOutWhenUnconnected=off
  Out2 : Outport  Port=2  VectorParamsAs1DForOutWhenUnconnected=off
  wires:
  SourceBlock/1 -> Out1/1
  SourceBlock/2 -> Out2/1

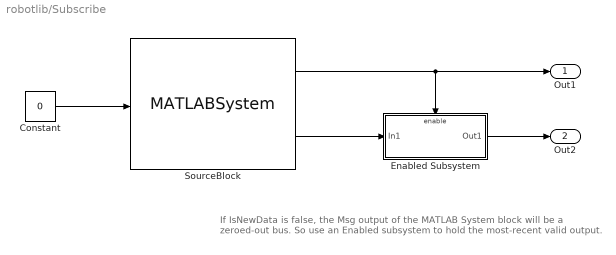
== system robotlib/Subscribe ==
  note: If IsNewData is false, the Msg output of the MATLAB System block will be a zeroed-out bus. So use an Enabled subsystem to hold the most-recent valid output.
  Constant : Constant  Value=0  VectorParams1D=off  OutDataTypeStr=Bus: SL_Bus_robotlib_geometry_msgs_Point  SampleTime=SampleTime  LockScale=on
  Enabled Subsystem : Subsystem  TreatAsAtomicUnit=on
  SourceBlock : MATLABSystem  System=ros.slroscpp.internal.block.Subscriber  MessageQueueLen=messageQueueLength  ROSTopic=/my_topic  ROSMessageType=geometry_msgs/Point  SLBusName=SL_Bus_robotlib_geometry_msgs_Point  ModelName=robotlib  BlockId=Sub_robotlib_93
      mask Type: ros.slroscpp.internal.block.Subscriber
  Out1 : Outport  VectorParamsAs1DForOutWhenUnconnected=off
  Out2 : Outport  Port=2  VectorParamsAs1DForOutWhenUnconnected=off  LockScale=on
  wires:
  Enabled Subsystem/1(Out1) -> Out2/1
  SourceBlock/2 -> Enabled Subsystem/1(In1)
  SourceBlock/1 -> Enabled Subsystem/Enable, Out1/1
  Constant/1 -> SourceBlock/1

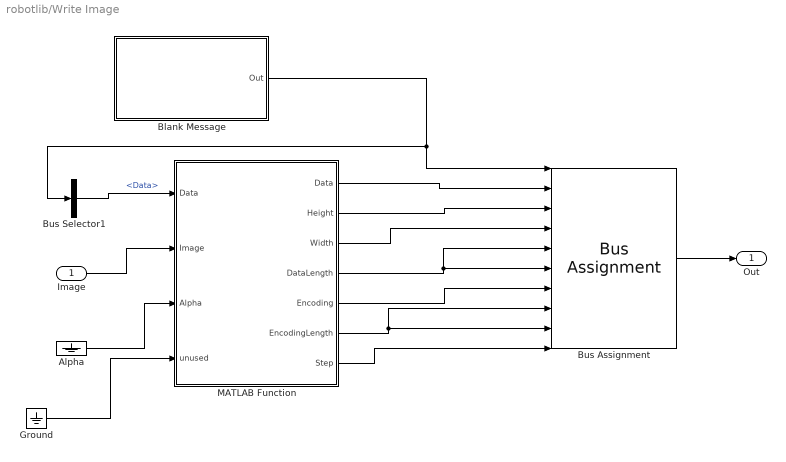
== system robotlib/Write Image ==
  Image : Inport
  Alpha : Ground
  Blank Message : Subsystem  LoadFcn=ros.slros.internal.block.MessageBlockMask.dispatch('loadFcn', gcb);  InitFcn=ros.slros.internal.block.errorIfBlocksConflict(bdroot(gcb));  TreatAsAtomicUnit=on  mask(ROS Blank Message){messageClass=Message, entityType=sensor_msgs/Image, messageType=sensor_msgs/Image, SampleTime=inf, legacyBusStruct=off}
      mask prompts: messageClass "ros:slros:blockmask:MessageClassPrompt"; entityType "ros:slros:blockmask:TypePrompt"; messageType "ros:slros:blockmask:FullTypePrompt"; SampleTime "Simulink:blkprm_prompts:AllSrcBlksSampleTime"; legacyBusStruct "Use legacy bus structure"
      mask help: ros:slros:blockmask:BlankMsgDescription
      mask init:
      | ros.slros.internal.block.MessageBlockMask.dispatch('maskInitialize', gcb);
      settings: ModelCloseFcn=ros.slros.internal.block.MessageBlockMask.dispatch('modelCloseFcn', gcb);  PreSaveFcn=ros.slros.internal.block.MessageBlockMask.dispatch('preSaveFcn', gcb);
      mask Help: eval('ros.slros.internal.helpview(''rosBlankMsgBlock'')');
      mask TypeOptions messageClass: ros:slros:blockmask:MessageType_Msg | ros:slros:blockmask:MessageType_SrvReq | ros:slros:blockmask:MessageType_SrvResp
      mask Callback messageClass: ros.slros.internal.block.MessageBlockMask.dispatch('messageClassChange', gcb);
      mask Callback entityType: ros.slros.internal.block.MessageBlockMask.dispatch('entityTypeEdit', gcb);
      mask TypeOptions SampleTime: Constant/SampleTime
      mask DialogControl messageClass Prompt: Class:
      mask DialogControl entityType Prompt: Type:
      mask DialogControl id_msgTypeSelectBtn Prompt: ros:slros:blockmask:SelectPrompt
      mask DialogControl id_msgTypeSelectBtn Callback: ros.slros.internal.block.MessageBlockMask.dispatch('selectButtonPressed', gcb);
      mask DialogControl messageType Prompt: Fully resolved type:
      mask DialogControl SampleTime Prompt: Sample time:
      mask Display: color('black');
  Bus Assignment : BusAssignment  AssignedSignals=Data,Height,Width,Data_SL_Info.CurrentLength,Data_SL_Info.ReceivedLength,Encoding,Encoding_SL_Info.CurrentLength,Encoding_SL_Info.ReceivedLength,Step
  Bus Selector1 : BusSelector  OutputSignals=Data
  Ground : Ground
  MATLAB Function : MATLAB Function  TreatAsAtomicUnit=on
  Out : Outport
  wires:
  MATLAB Function/3(Width) -> Bus Assignment/4
  Alpha/1 -> MATLAB Function/3(Alpha)
  MATLAB Function/1(Data) -> Bus Assignment/2
  MATLAB Function/5(Encoding) -> Bus Assignment/7
  Bus Selector1/1 -> MATLAB Function/1("Data ")  "<Data>"
  MATLAB Function/7(Step) -> Bus Assignment/10
  MATLAB Function/4(DataLength) -> Bus Assignment/6, Bus Assignment/5
  Bus Assignment/1 -> Out/1
  MATLAB Function/6(EncodingLength) -> Bus Assignment/9, Bus Assignment/8
  Ground/1 -> MATLAB Function/4(unused)
  Image/1 -> MATLAB Function/2(Image)
  Blank Message/1(Out) -> Bus Assignment/1, Bus Selector1/1
  MATLAB Function/2(Height) -> Bus Assignment/3

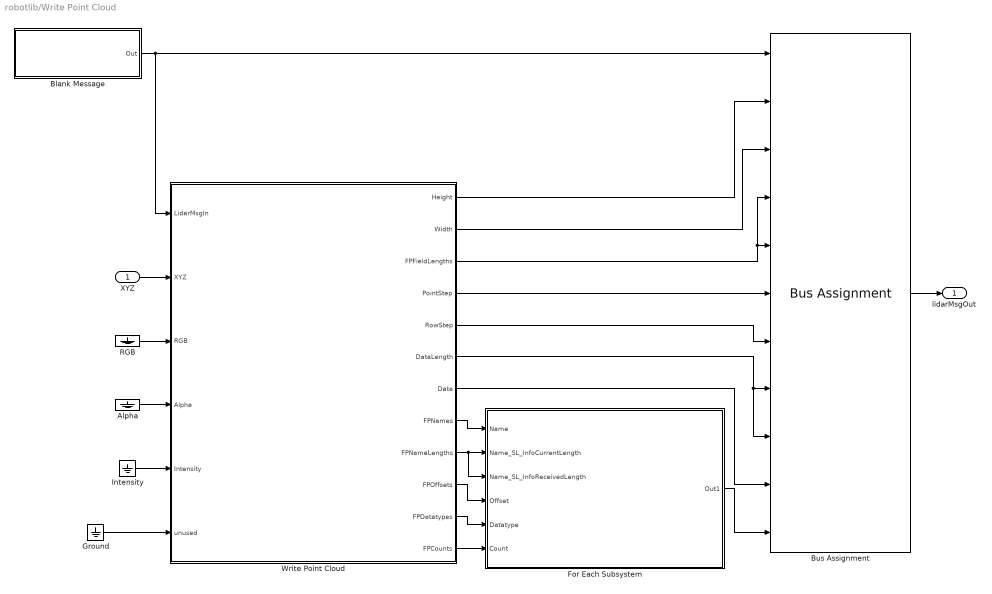
== system robotlib/Write Point Cloud ==
  XYZ : Inport
  Alpha : Ground
  Blank Message : Subsystem  LoadFcn=ros.slros.internal.block.MessageBlockMask.dispatch('loadFcn', gcb);  InitFcn=ros.slros.internal.block.errorIfBlocksConflict(bdroot(gcb));  TreatAsAtomicUnit=on  mask(ROS Blank Message){messageClass=Message, entityType=sensor_msgs/PointCloud2, messageType=sensor_msgs/PointCloud2, SampleTime=inf, legacyBusStruct=off}
      mask prompts: messageClass "ros:slros:blockmask:MessageClassPrompt"; entityType "ros:slros:blockmask:TypePrompt"; messageType "ros:slros:blockmask:FullTypePrompt"; SampleTime "Simulink:blkprm_prompts:AllSrcBlksSampleTime"; legacyBusStruct "Use legacy bus structure"
      mask help: ros:slros:blockmask:BlankMsgDescription
      mask init:
      | ros.slros.internal.block.MessageBlockMask.dispatch('maskInitialize', gcb);
      settings: ModelCloseFcn=ros.slros.internal.block.MessageBlockMask.dispatch('modelCloseFcn', gcb);  PreSaveFcn=ros.slros.internal.block.MessageBlockMask.dispatch('preSaveFcn', gcb);
      mask Help: eval('ros.slros.internal.helpview(''rosBlankMsgBlock'')');
      mask TypeOptions messageClass: ros:slros:blockmask:MessageType_Msg | ros:slros:blockmask:MessageType_SrvReq | ros:slros:blockmask:MessageType_SrvResp
      mask Callback messageClass: ros.slros.internal.block.MessageBlockMask.dispatch('messageClassChange', gcb);
      mask Callback entityType: ros.slros.internal.block.MessageBlockMask.dispatch('entityTypeEdit', gcb);
      mask TypeOptions SampleTime: Constant/SampleTime
      mask DialogControl messageClass Prompt: Class:
      mask DialogControl entityType Prompt: Type:
      mask DialogControl id_msgTypeSelectBtn Prompt: ros:slros:blockmask:SelectPrompt
      mask DialogControl id_msgTypeSelectBtn Callback: ros.slros.internal.block.MessageBlockMask.dispatch('selectButtonPressed', gcb);
      mask DialogControl messageType Prompt: Fully resolved type:
      mask DialogControl SampleTime Prompt: Sample time:
      mask Display: color('black');
  Bus Assignment : BusAssignment  AssignedSignals=Height,Width,Fields_SL_Info.CurrentLength,Fields_SL_Info.ReceivedLength,PointStep,RowStep,Data_SL_Info.CurrentLength,Data_SL_Info.ReceivedLength,Data,Fields
  For Each Subsystem : Subsystem  TreatAsAtomicUnit=on
  Ground : Ground
  Intensity : Ground
  RGB : Ground
  Write Point Cloud : MATLAB Function  TreatAsAtomicUnit=on
  lidarMsgOut : Outport
  wires:
  Ground/1 -> Write Point Cloud/6(unused)
  Blank Message/1(Out) -> Bus Assignment/1, Write Point Cloud/1(LidarMsgIn)
  Write Point Cloud/6(DataLength) -> Bus Assignment/8, Bus Assignment/9
  Write Point Cloud/12(FPCounts) -> For Each Subsystem/6(Count)
  Write Point Cloud/4(PointStep) -> Bus Assignment/6
  RGB/1 -> Write Point Cloud/3(RGB)
  Write Point Cloud/8(FPNames) -> For Each Subsystem/1(Name)
  Write Point Cloud/7(Data) -> Bus Assignment/10
  Write Point Cloud/1(Height) -> Bus Assignment/2
  Write Point Cloud/9(FPNameLengths) -> For Each Subsystem/2(Name_SL_InfoCurrentLength), For Each Subsystem/3(Name_SL_InfoReceivedLength)
  Write Point Cloud/11(FPDatatypes) -> For Each Subsystem/5(Datatype)
  Write Point Cloud/3(FPFieldLengths) -> Bus Assignment/4, Bus Assignment/5
  For Each Subsystem/1(Out1) -> Bus Assignment/11
  Write Point Cloud/10(FPOffsets) -> For Each Subsystem/4(Offset)
  Write Point Cloud/2(Width) -> Bus Assignment/3
  Write Point Cloud/5(RowStep) -> Bus Assignment/7
  XYZ/1 -> Write Point Cloud/2(XYZ)
  Bus Assignment/1 -> lidarMsgOut/1
  Alpha/1 -> Write Point Cloud/4(Alpha)
  Intensity/1 -> Write Point Cloud/5(Intensity)

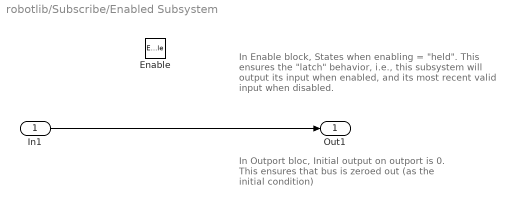
== system robotlib/Subscribe/Enabled Subsystem ==
  note: In Outport bloc, Initial output on outport is 0.
      | This ensures that bus is zeroed out
      | (as the initial condition)
  note: In Enable block, States when enabling = "held".
      | This ensures the "latch" behavior, i.e., this subsystem
      | will output its input when enabled, and its most recent
      | valid input when disabled.
  In1 : Inport
  Enable : EnablePort
  Out1 : Outport  InitialOutput=0  VectorParamsAs1DForOutWhenUnconnected=off
  wires:
  In1/1 -> Out1/1

== system robotlib/Write Image/Blank Message ==
  Constant : Constant  InitFcn=ros.slros.internal.block.MessageBlockMask.dispatch('constantBlkInitFcn', gcb);  Value=0  OutDataTypeStr=Bus: SL_Bus_robotlib_sensor_msgs_Image  SampleTime=SampleTime  LockScale=on
  Out : Outport  VectorParamsAs1DForOutWhenUnconnected=off  LockScale=on
  wires:
  Constant/1 -> Out/1

== system robotlib/Write Point Cloud/Blank Message ==
  Constant : Constant  InitFcn=ros.slros.internal.block.MessageBlockMask.dispatch('constantBlkInitFcn', gcb);  Value=0  OutDataTypeStr=Bus: SL_Bus_write_point_cloud_example_PointCloud2_hs0618  SampleTime=SampleTime  LockScale=on
  Out : Outport  VectorParamsAs1DForOutWhenUnconnected=off  LockScale=on
  wires:
  Constant/1 -> Out/1

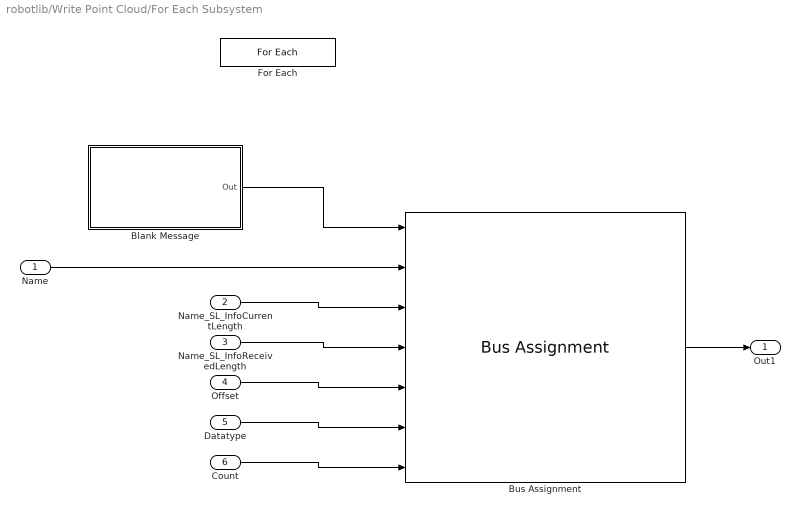
== system robotlib/Write Point Cloud/For Each Subsystem ==
  Name : Inport  Partition=on  PartitionDimension=1  PartitionWidth=ros.slros.internal.bus.Util.getCurrentFieldLength('sensor_msgs/PointField','Name','ros')  PartitionOffset=0
  Name_SL_InfoCurrentLength : Inport  Port=2  Partition=on  PartitionDimension=1  PartitionWidth=1  PartitionOffset=0
  Name_SL_InfoReceivedLength : Inport  Port=3  Partition=on  PartitionDimension=1  PartitionWidth=1  PartitionOffset=0
  Offset : Inport  Port=4  Partition=on  PartitionDimension=1  PartitionWidth=1  PartitionOffset=0
  Datatype : Inport  Port=5  Partition=on  PartitionDimension=1  PartitionWidth=1  PartitionOffset=0
  Count : Inport  Port=6  Partition=on  PartitionDimension=1  PartitionWidth=1  PartitionOffset=0
  Blank Message : Subsystem  LoadFcn=ros.slros.internal.block.MessageBlockMask.dispatch('loadFcn', gcb);  InitFcn=ros.slros.internal.block.errorIfBlocksConflict(bdroot(gcb));  TreatAsAtomicUnit=on  mask(ROS Blank Message){messageClass=Message, entityType=sensor_msgs/PointField, messageType=sensor_msgs/PointField, SampleTime=inf, legacyBusStruct=off}
      mask prompts: messageClass "ros:slros:blockmask:MessageClassPrompt"; entityType "ros:slros:blockmask:TypePrompt"; messageType "ros:slros:blockmask:FullTypePrompt"; SampleTime "Simulink:blkprm_prompts:AllSrcBlksSampleTime"; legacyBusStruct "Use legacy bus structure"
      mask help: ros:slros:blockmask:BlankMsgDescription
      mask init:
      | ros.slros.internal.block.MessageBlockMask.dispatch('maskInitialize', gcb);
      settings: ModelCloseFcn=ros.slros.internal.block.MessageBlockMask.dispatch('modelCloseFcn', gcb);  PreSaveFcn=ros.slros.internal.block.MessageBlockMask.dispatch('preSaveFcn', gcb);
      mask Help: eval('ros.slros.internal.helpview(''rosBlankMsgBlock'')');
      mask TypeOptions messageClass: ros:slros:blockmask:MessageType_Msg | ros:slros:blockmask:MessageType_SrvReq | ros:slros:blockmask:MessageType_SrvResp
      mask Callback messageClass: ros.slros.internal.block.MessageBlockMask.dispatch('messageClassChange', gcb);
      mask Callback entityType: ros.slros.internal.block.MessageBlockMask.dispatch('entityTypeEdit', gcb);
      mask TypeOptions SampleTime: Constant/SampleTime
      mask DialogControl messageClass Prompt: Class:
      mask DialogControl entityType Prompt: Type:
      mask DialogControl id_msgTypeSelectBtn Prompt: ros:slros:blockmask:SelectPrompt
      mask DialogControl id_msgTypeSelectBtn Callback: ros.slros.internal.block.MessageBlockMask.dispatch('selectButtonPressed', gcb);
      mask DialogControl messageType Prompt: Fully resolved type:
      mask DialogControl SampleTime Prompt: Sample time:
      mask Display: color('black');
  Bus Assignment : BusAssignment  AssignedSignals=Name,Name_SL_Info.CurrentLength,Name_SL_Info.ReceivedLength,Offset,Datatype,Count
  For Each : ForEach  DisableCoverage=on
  Out1 : Outport  ConcatenationDimension=1
  wires:
  Name/1 -> Bus Assignment/2
  Count/1 -> Bus Assignment/7
  Datatype/1 -> Bus Assignment/6
  Offset/1 -> Bus Assignment/5
  Name_SL_InfoReceivedLength/1 -> Bus Assignment/4
  Name_SL_InfoCurrentLength/1 -> Bus Assignment/3
  Bus Assignment/1 -> Out1/1
  Blank Message/1(Out) -> Bus Assignment/1

== system robotlib/Write Point Cloud/For Each Subsystem/Blank Message ==
  Constant : Constant  InitFcn=ros.slros.internal.block.MessageBlockMask.dispatch('constantBlkInitFcn', gcb);  Value=0  OutDataTypeStr=Bus: SL_Bus_write_point_cloud_example_PointField_2wq1bf  SampleTime=SampleTime  LockScale=on
  Out : Outport  VectorParamsAs1DForOutWhenUnconnected=off  LockScale=on
  wires:
  Constant/1 -> Out/1

== matlab function robotlib/Write Point Cloud/Write Point Cloud ==
  data: LidarMsgIn input; XYZ input; RGB input; Alpha input; Intensity input; unused input; FieldNamesStruct parameter; HasRGB parameter; HasAlpha parameter; Height output; Width output; FPFieldLengths output; PointStep output; RowStep output; DataLength output; Data output; FPNames output; FPNameLengths output; FPOffsets output; FPDatatypes output; FPCounts output; HasIntensity parameter
function [Height, Width, FPFieldLengths, PointStep, ...
    RowStep, DataLength, Data, FPNames,...
    FPNameLengths, FPOffsets, FPDatatypes, FPCounts] ...
    = WritePointCloudFcnBlock(LidarMsgIn, XYZ, RGB, Alpha, Intensity, ~,...
    FieldNamesStruct, HasRGB, HasAlpha, HasIntensity)

unstructured = ismatrix(XYZ); 

MaxDataLength = length(LidarMsgIn.Data);
NumFields = length(LidarMsgIn.Fields);
NameLength = length(LidarMsgIn.Fields(1).Name);

[Height, Width, FPFieldLengths, PointStep, RowStep, DataLength, Data,   ...
    FPNames, FPNameLengths, FPOffsets, FPDatatypes, FPCounts] =         ...
    ros.internal.block.WritePointCloudFcnBlock(MaxDataLength, NumFields,...
    NameLength, XYZ, RGB, Alpha, Intensity, unstructured, HasRGB,       ...
    HasAlpha, HasIntensity, FieldNamesStruct, 'ROS');
